simulink model "Flight_Sim"  (R2023a)
settings: Solver=VariableStepAuto  StartTime=0.0  StopTime=10  RelTol=1e-3
values from neighbouring files (symbols this model uses):
  sigma_c = 8.60002996569e-06    [Roll_variables.mat]
  sigma_f = 2.2194295764e-05    [Roll_variables.mat]
settings Model: Creator=kwood  LastModifiedBy=A-0001
settings DebuggingCC: ModelReferenceExtraNoncontSigs=none

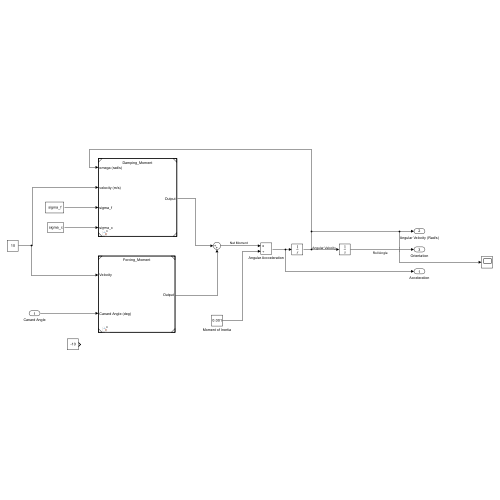
[thumbnail: Simulink's stored preview of the top-level diagram]
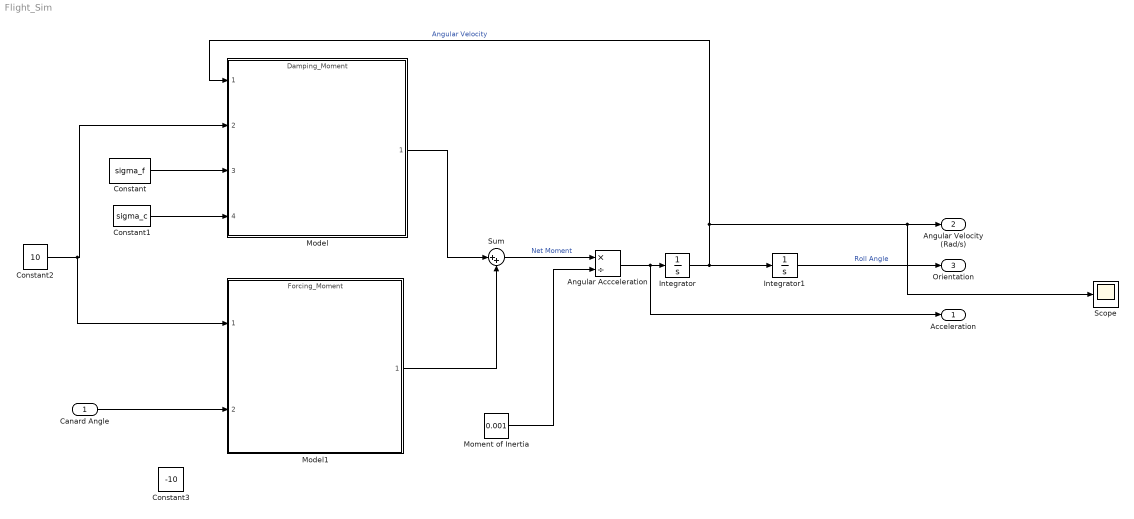
== system Flight_Sim ==
  Canard Angle : Inport
  Angular Accceleration : Product  Inputs=*/
  Constant : Constant  Value=sigma_f
  Constant1 : Constant  Value=sigma_c
  Constant2 : Constant  Value=10
  Constant3 : Constant  Value=-10
  Integrator : Integrator
  Integrator1 : Integrator
  Model : ModelReference  ModelNameDialog=Damping_Moment.slx  SimulationMode=Normal  ModelReferenceVersion=1.3
  Model1 : ModelReference  ModelNameDialog=Forcing_Moment.slx  SimulationMode=Normal  ModelReferenceVersion=1.2
  Moment of Inertia : Constant  Value=0.001
  Scope : Scope
  Sum : Sum  Inputs=|++
  Acceleration : Outport
  Angular Velocity (Rad/s) : Outport  Port=2
  Orientation : Outport  Port=3
  wires:
  Model1/1 -> Sum/2
  Sum/1 -> Angular Accceleration/1  "Net Moment"
  Integrator/1 -> Integrator1/1, Model/1, Scope/1, Angular Velocity (Rad/s)/1  "Angular Velocity"
  Constant2/1 -> Model1/1, Model/2
  Moment of Inertia/1 -> Angular Accceleration/2
  Angular Accceleration/1 -> Acceleration/1, Integrator/1
  Integrator1/1 -> Orientation/1  "Roll Angle"
  Canard Angle/1 -> Model1/2
  Model/1 -> Sum/1
  Constant/1 -> Model/3
  Constant1/1 -> Model/4
